simulink model "unlinear_model"  (R2024b)
settings: Solver=VariableStepAuto  StartTime=0.0  StopTime=30  RelTol=1e-3
undefined symbols (not defined in the file): K
settings Model: Creator=O5-3  LastModifiedBy=norbe

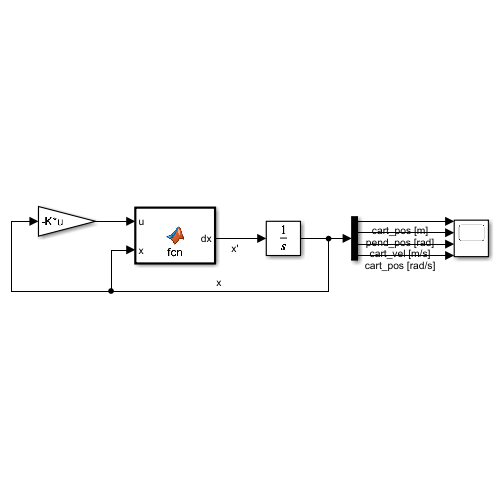
[thumbnail: Simulink's stored preview of the top-level diagram]
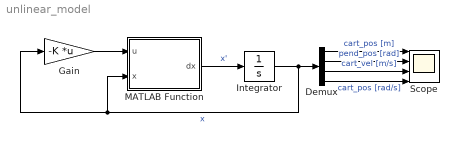
== system unlinear_model ==
  Demux : Demux
  Gain : Gain  Gain=-K  Multiplication=Matrix(K*u)
  Integrator : Integrator  InitialCondition=[-0.5;0.10;0;0]
  MATLAB Function : MATLAB Function  TreatAsAtomicUnit=on
  Scope : Scope  NumInputPorts=4
  wires:
  MATLAB Function/1(dx) -> Integrator/1  "x'"
  Gain/1 -> MATLAB Function/1(u)
  Integrator/1 -> Demux/1, Gain/1, MATLAB Function/2(x)  "x"
  Demux/1 -> Scope/1  "cart_pos [m]"
  Demux/2 -> Scope/2  "pend_pos [rad]"
  Demux/3 -> Scope/3  "cart_vel [m/s]"
  Demux/4 -> Scope/4  "cart_pos [rad/s]"

== matlab function unlinear_model/MATLAB Function ==
  data: u input; dx output; x input
function dx = fcn(u, x)

x2 = x(2);
x3 = x(3);
x4 = x(4);

fc = 1.88;
fp = 2.6465e-4;
l = 0.0492;
g = 9.81;
J = 0.0132;
mc = 0.605;
mp = 0.088;
a = l^2+J/(mc+mp);
mi = l*(mc+mp);

d1 = x3;
d2 = x4;
d3 = (a*(u-mi*(x4^2)*sin(x2)-fc*x3)+l*cos(x2)*(mi*g*sin(x2)-fp*x4))/(J-mi*l*cos(x2)^2);
d4 = (l*cos(x2)*(u-mi*(x4^2)*sin(x2)-fc*x3)+mi*g*sin(x2)-fp*x4)/(J-mi*l*cos(x2)^2);

dx = [d1;d2;d3;d4];
